simulink library "adrc_toolbox_library_2021"  (R2021a)
settings: Solver=VariableStepAuto  StartTime=0.0  StopTime=10.0  RelTol=1e-3
settings Model: Creator=krzys  LastModifiedBy=krzys

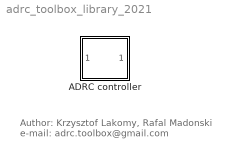
== system adrc_toolbox_library_2021 ==
  note: Author: Krzysztof Lakomy, Rafal Madonski
      | e-mail: adrc.toolbox@gmail.com
  ADRC controller : Subsystem  mask(ADRC controller){dynamicsOrder=2, controllerBandwidth=5, controllerBandwidthSource=Internal, observerBandwidth=25, observerBandwidthSource=Internal, inputGainParameter=1, inputGainSource=Internal, saturationEnabled=on, UpperLimit=10, LowerLimit=-10, deadTimeEnabled=off, deadTime=0.2}
      mask prompts: dynamicsOrder "Dynamics order (n):"; controllerBandwidth "Value [rad/s]:"; controllerBandwidthSource "Source:"; observerBandwidth "Value [rad/s]:"; observerBandwidthSource "Source:"; inputGainParameter "Value:"; inputGainSource "Source:"; saturationEnabled "Saturation"; UpperLimit "Upper limit (u_max):"; LowerLimit "Lower limit (u_min):"; deadTimeEnabled "Anti-peaking"; deadTime "Controller start time [s] (T_d):"
      mask help: The ADRC controller is a part of the Active Disturbance Rejection Control (ADRC) Toolbox, available at: https://www.mathworks.com/matlabcentral/fileexchange/102249-active-disturbance-rejection-control-adrc-toolbox
      mask init:
      | set_param(gcb,'MaskHideContents','off');
      | set_param(gcb, 'MaskSelfModifiable', 'on');
      | 
      | controllerBandwidthSource = get_param(gcb,'controllerBandwidthSource');
      | switch(controllerBandwidthSource)
      |     case 'Internal'
      |         replace_block([gcb,'/controllerBandwidthIn'], 'Inport', 'Ground', 'noprompt');
      |         inputGainParameterType = 'Internal';
      |     case 'External'
      |         replace_block([gcb,'/controllerBandwidthIn'], 'Ground', 'Inport', 'noprompt');
      |         inputGainParameterType = 'External';
      | end
      | 
      | observerBandwidthSource = get_param(gcb,'observerBandwidthSource');
      | switch(observerBandwidthSource)
      |     case 'Internal'
      |         replace_block([gcb,'/observerBandwidthIn'], 'Inport', 'Ground', 'noprompt');
      |         inputGainParameterType = 'Internal';
      |     case 'External'
      |         replace_block([gcb,'/observerBandwidthIn'], 'Ground', 'Inport', 'noprompt');
      |         inputGainParameterType = 'External';
      | end
      | 
      | inputGainSource = get_param(gcb,'inputGainSource');
      | switch(inputGainSource)
      |     case 'Internal'
      |         replace_block([gcb,'/inputGainParameterIn'], 'Inport', 'Ground', 'noprompt');
      |         inputGainParameterType = 'Internal';
      |     case 'External'
      |         replace_block([gcb,'/inputGainParameterIn'], 'Ground', 'Inport', 'noprompt');
      |         inputGainParameterType = 'External';
      | end
      mask Help:
      | The ADRC controller is a single, drag-and-drop, Simulink function block that encapsulates a specific continous-time error-based active disturbance rejection control (ADRC) algorithm. For simplicity and compactness, the ADRC controller is developed as a single input (feedback error signal), single output (control signal) block, which can be used as a powerful alternative to the conventional PID controller.
      | 
      | The design parameters of the implemented ADRC algorithm can be easily changed using the provided graphical user interface (GUI). The GUI also allows to activate two practical functionalities, namely: saturation of the control signal and anti-peaking mechanism.
      | 
      | The ADRC controller is a part of the Active Disturbance Rejection Control (ADRC) Toolbox. The goal of the Active Disturbance Rejection Control (ADRC) Toolbox is to provide an intuitive contol solution for Simulink, allowing to implement the ADRC algorithm in simulations/experiments quickly and with low effort.
      | 
      | Code contributors: Krzysztof Lakomy, Rafal Madonski, Jacek Michalski, Wojciech Giernacki
      | 
      | Contact: adrc.toolbox@gmail.com
      | 
      | More information at: https://www.mathworks.com/matlabcentral/fileexchange/102249-active-disturbance-rejection-control-adrc-toolbox
      mask TypeOptions dynamicsOrder: Linear extended state observer/dynamicsOrder | State feedback robust controller/dynamicsOrder
      mask TypeOptions controllerBandwidth: State feedback robust controller/controllerBandwidth
      mask TypeOptions controllerBandwidthSource: Internal | External
      mask Callback controllerBandwidthSource:
      | controllerBandwidthSource = get_param(gcb,'controllerBandwidthSource');
      | en = get_param(gcb,'MaskEnables');
      | 
      | switch(controllerBandwidthSource)
      |     case 'Internal'
      |         en{2} = 'on';
      |     case 'External'
      |         en{2} = 'off';
      | end
      | 
      | set_param(gcb,'MaskEnables',en);
      mask TypeOptions observerBandwidth: Linear extended state observer/observerBandwidth
      mask TypeOptions observerBandwidthSource: Internal | External
      mask Callback observerBandwidthSource:
      | observerBandwidthSource = get_param(gcb,'observerBandwidthSource');
      | en = get_param(gcb,'MaskEnables');
      | 
      | switch(observerBandwidthSource)
      |     case 'Internal'
      |         en{4} = 'on';
      |     case 'External'
      |         en{4} = 'off';
      | end
      | 
      | set_param(gcb,'MaskEnables',en);
      mask TypeOptions inputGainParameter: Linear extended state observer/inputGainParameter | State feedback robust controller/inputGainParameter
      mask TypeOptions inputGainSource: Internal | External
      mask Callback inputGainSource:
      | inputGainSource = get_param(gcb,'inputGainSource');
      | en = get_param(gcb,'MaskEnables');
      | 
      | switch(inputGainSource)
      |     case 'Internal'
      |         en{6} = 'on';
      |     case 'External'
      |         en{6} = 'off';
      | end
      | 
      | set_param(gcb,'MaskEnables',en);
      mask TypeOptions saturationEnabled: State feedback robust controller/saturationEnabled
      mask Callback saturationEnabled:
      | saturationEnabled = get_param(gcb,'saturationEnabled');
      | en = get_param(gcb,'MaskEnables');
      | 
      | switch(saturationEnabled)
      |     case 'on'
      |         en{9} = 'on';
      |         en{10} = 'on';
      |     case 'off'
      |         en{9} = 'off';
      |         en{10} = 'off';
      | end
      | 
      | set_param(gcb,'MaskEnables',en);
      mask TypeOptions UpperLimit: State feedback robust controller/UpperLimit
      mask TypeOptions LowerLimit: State feedback robust controller/LowerLimit
      mask TypeOptions deadTimeEnabled: State feedback robust controller/deadTimeEnabled
      mask Callback deadTimeEnabled:
      | deadTimeEnabled = get_param(gcb,'deadTimeEnabled');
      | en = get_param(gcb,'MaskEnables');
      | 
      | switch(deadTimeEnabled)
      |     case 'on'
      |         en{12} = 'on';
      |     case 'off'
      |         en{12} = 'off';
      | end
      | 
      | set_param(gcb,'MaskEnables',en);
      mask TypeOptions deadTime: State feedback robust controller/Time
      mask DialogControl DescGroupVar Prompt: Active Disturbance Rejection Controller (ADRC)
      mask DialogControl DescTextVar Prompt: This block implements an error-based continuous-time Active Disturbance Rejection Controller (ADRC). The default form of this controller calculates the control signal (block output) based only on the control feedback error (block input).
      mask DialogControl ParameterGroupVar Prompt: Control system parameters
      mask DialogControl Container5 Prompt: Parameters
      mask DialogControl Container12 Prompt: Controller bandwidth (omega_c):
      mask DialogControl Container11 Prompt: Observer bandwidth (omega_o):
      mask DialogControl Container10 Prompt: Input gain (b_hat):
      mask DialogControl Container4 Prompt: Saturation
      mask DialogControl Control3 Prompt: Saturation functionality limits the boundary values of the control signal, allowing to adjust the output of the ADRC controller block to the physical limitations of the controlled system.
      mask DialogControl Container8 Prompt: Anti-peaking
      mask DialogControl Control4 Prompt: Anti-peaking functionality is obtained by delaying the controller start by a specified time value (in seconds), allowing the observer transient state to pass.
      mask Display:
      | inputGainSource = get_param(gcb,'inputGainSource');
      | observerBandwidthSource = get_param(gcb,'observerBandwidthSource');
      | controllerBandwidthSource = get_param(gcb,'controllerBandwidthSource');
      | 
      | disp('ADRC');
      | switch controllerBandwidthSource
      |     case 'Internal'
      |     case 'External'
      |         port_label('input',1,'e');
      |         port_label('input',2,'wc');
      | end
      | switch observerBandwidthSource
      |     case 'Internal'
      |     case 'External'
      |         port_label('input',1,'e');
      |         if(strcmp(controllerBandwidthSource,'External'))
      |             port_label('input',3,'wo');
      |         else
      |             port_label('input',2,'wo');
      |         end
      | end
      | switch inputGainSource
      |     case 'Internal'
      |     case 'External'
      |         port_label('input',1,'e');
      |         if(strcmp(controllerBandwidthSource,'External') && strcmp(observerBandwidthSource,'External'))
      |             port_label('input',4,'b');
      |         elseif(xor(strcmp(controllerBandwidthSource,'External'), strcmp(observerBandwidthSource,'External')))
      |             port_label('input',3,'b');
      |         else
      |             port_label('input',2,'b');
      |         end
      | end

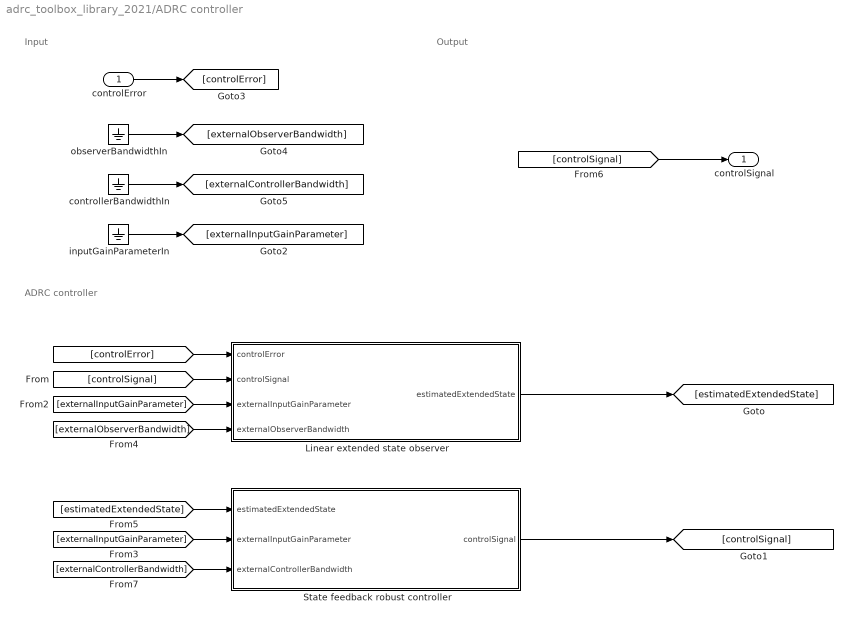
== system adrc_toolbox_library_2021/ADRC controller ==
  note: ADRC controller
  note: Output
  note: Input
  controlError : Inport
  Linear extended state observer : Subsystem  mask{InitialCondition=zeros(dynamicsOrder+1,1), dynamicsOrder=dynamicsOrder, observerBandwidth=observerBandwidth, inputGainParameter=inputGainParameter}
      mask prompts: InitialCondition "Integrator initial conditions:"; dynamicsOrder "Dynamics order:"; observerBandwidth "Observer bandwidth:"; inputGainParameter "Input gain parameter:"
      mask TypeOptions InitialCondition: Integrator/InitialCondition
      mask TypeOptions dynamicsOrder: Linear extended state observer/dynamicsOrder
      mask TypeOptions observerBandwidth: Linear extended state observer/observerBandwidth
      mask TypeOptions inputGainParameter: Linear extended state observer/inputGainParameter
  State feedback robust controller : Subsystem  mask{dynamicsOrder=dynamicsOrder, inputGainParameter=inputGainParameter, controllerBandwidth=controllerBandwidth, saturationEnabled=on, UpperLimit=UpperLimit, LowerLimit=LowerLimit, deadTimeEnabled=off, Time=deadTime}
      mask prompts: dynamicsOrder "Dynamics order:"; inputGainParameter "Input gain parameter:"; controllerBandwidth "Controller bandwidth:"; saturationEnabled "Output saturation"; UpperLimit "Simulink:blkprm_prompts:SaturateUpLim"; LowerLimit "Simulink:blkprm_prompts:SaturateLowLim"; deadTimeEnabled "Dead time enabled"; Time "Dead time:"
      mask TypeOptions dynamicsOrder: Extended state feedback robust controller/dynamicsOrder
      mask TypeOptions inputGainParameter: Extended state feedback robust controller/inputGainParameter
      mask TypeOptions controllerBandwidth: Extended state feedback robust controller/controllerBandwidth
      mask TypeOptions saturationEnabled: Saturation/saturationEnabled
      mask TypeOptions UpperLimit: Saturation/UpperLimit
      mask TypeOptions LowerLimit: Saturation/LowerLimit
      mask TypeOptions deadTimeEnabled: Dead time/deadTimeEnabled
      mask TypeOptions Time: Dead time/Time
      mask DialogControl UpperLimit Prompt: Upper limit:
      mask DialogControl LowerLimit Prompt: Lower limit:
  controllerBandwidthIn : Ground
  inputGainParameterIn : Ground
  observerBandwidthIn : Ground
  controlSignal : Outport
  wires:
  [controlSignal] -> controlSignal/1
  [controlError] -> Linear extended state observer/1(controlError)
  [controlSignal] -> Linear extended state observer/2(controlSignal)
  controlError/1 -> [controlError]
  Linear extended state observer/1(estimatedExtendedState) -> [estimatedExtendedState]
  [estimatedExtendedState] -> State feedback robust controller/1(estimatedExtendedState)
  inputGainParameterIn/1 -> [externalInputGainParameter]
  [externalInputGainParameter] -> Linear extended state observer/3(externalInputGainParameter)
  [externalInputGainParameter] -> State feedback robust controller/2(externalInputGainParameter)
  State feedback robust controller/1(controlSignal) -> [controlSignal]
  observerBandwidthIn/1 -> [externalObserverBandwidth]
  [externalObserverBandwidth] -> Linear extended state observer/4(externalObserverBandwidth)
  controllerBandwidthIn/1 -> [externalControllerBandwidth]
  [externalControllerBandwidth] -> State feedback robust controller/3(externalControllerBandwidth)

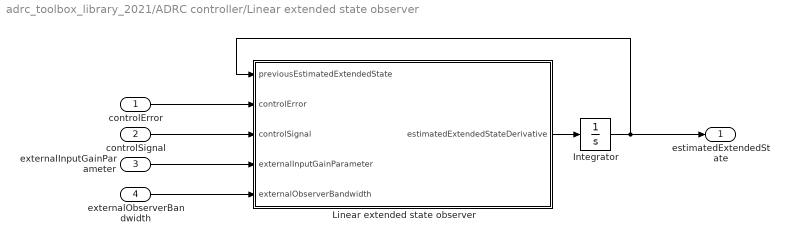
== system adrc_toolbox_library_2021/ADRC controller/Linear extended state observer ==
  controlError : Inport
  controlSignal : Inport  Port=2
  externalInputGainParameter : Inport  Port=3  PortDimensions=1
  externalObserverBandwidth : Inport  Port=4  PortDimensions=1
  Integrator : Integrator  InitialCondition=InitialCondition
  Linear extended state observer : MATLAB Function  TreatAsAtomicUnit=on  mask{dynamicsOrder=dynamicsOrder, observerBandwidth=observerBandwidth, inputGainParameter=inputGainParameter}
      mask prompts: dynamicsOrder "Dynamics order:"; observerBandwidth "Observer bandwidth:"; inputGainParameter "Input gain parameter:"
  estimatedExtendedState : Outport
  wires:
  controlError/1 -> Linear extended state observer/2(controlError)
  Linear extended state observer/1(estimatedExtendedStateDerivative) -> Integrator/1
  externalInputGainParameter/1 -> Linear extended state observer/4(externalInputGainParameter)
  controlSignal/1 -> Linear extended state observer/3(controlSignal)
  Integrator/1 -> Linear extended state observer/1(previousEstimatedExtendedState), estimatedExtendedState/1
  externalObserverBandwidth/1 -> Linear extended state observer/5(externalObserverBandwidth)

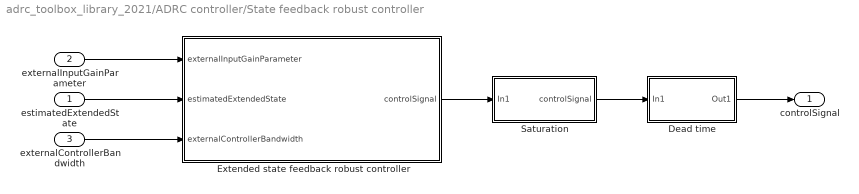
== system adrc_toolbox_library_2021/ADRC controller/State feedback robust controller ==
  estimatedExtendedState : Inport  PortDimensions=dynamicsOrder+1
  externalInputGainParameter : Inport  Port=2  PortDimensions=1  SampleTime=1
  externalControllerBandwidth : Inport  Port=3  PortDimensions=1
  Dead time : Subsystem  Variant=on  VariantControlMode=label  LabelModeActiveChoice=dead_time_off  mask{deadTimeEnabled=off, Time=Time}
      mask prompts: deadTimeEnabled "Dead time enabled"; Time "Dead time:"
      mask Callback deadTimeEnabled:
      | deadTimeChoice = get_param(gcb,'deadTimeEnabled');
      | if strcmp(deadTimeChoice,'off')
      |     set_param(gcb, 'LabelModeActiveChoice', 'dead_time_off');
      | else
      |     set_param(gcb, 'LabelModeActiveChoice', 'dead_time_on');
      | end
      mask TypeOptions Time: Dead time on/Step/Time
  Extended state feedback robust controller : MATLAB Function  TreatAsAtomicUnit=on  mask{dynamicsOrder=dynamicsOrder, inputGainParameter=inputGainParameter, controllerBandwidth=controllerBandwidth}
      mask prompts: dynamicsOrder "Dynamics order:"; inputGainParameter "Input gain parameter:"; controllerBandwidth "Controller bandwidth:"
  Saturation : Subsystem  Variant=on  VariantControlMode=label  LabelModeActiveChoice=saturation_off  mask{saturationEnabled=on, UpperLimit=UpperLimit, LowerLimit=LowerLimit}
      mask prompts: saturationEnabled "Output saturation"; UpperLimit "Simulink:blkprm_prompts:SaturateUpLim"; LowerLimit "Simulink:blkprm_prompts:SaturateLowLim"
      mask Callback saturationEnabled:
      | saturationChoice = get_param(gcb,'saturationEnabled');
      | if strcmp(saturationChoice,'off')
      |     set_param(gcb, 'LabelModeActiveChoice', 'saturation_off');
      | else
      |     set_param(gcb, 'LabelModeActiveChoice', 'saturation_on');
      | end
      mask TypeOptions UpperLimit: Saturation on/Saturation/UpperLimit
      mask TypeOptions LowerLimit: Saturation on/Saturation/LowerLimit
      mask DialogControl UpperLimit Prompt: Upper limit:
      mask DialogControl LowerLimit Prompt: Lower limit:
  controlSignal : Outport
  wires:
  estimatedExtendedState/1 -> Extended state feedback robust controller/2(estimatedExtendedState)
  externalInputGainParameter/1 -> Extended state feedback robust controller/1(externalInputGainParameter)
  Extended state feedback robust controller/1(controlSignal) -> Saturation/1(In1)
  externalControllerBandwidth/1 -> Extended state feedback robust controller/3(externalControllerBandwidth)
  Saturation/1(controlSignal) -> Dead time/1(In1)
  Dead time/1(Out1) -> controlSignal/1

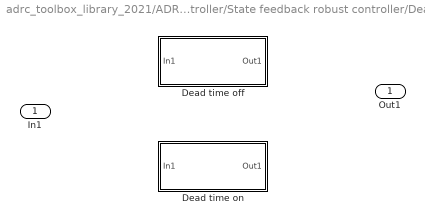
== system adrc_toolbox_library_2021/ADRC controller/State feedback robust controller/Dead time ==
  In1 : Inport
  Dead time off : Subsystem  VariantControl=dead_time_off
  Dead time on : Subsystem  VariantControl=dead_time_on
  Out1 : Outport

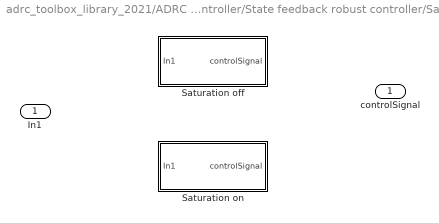
== system adrc_toolbox_library_2021/ADRC controller/State feedback robust controller/Saturation ==
  In1 : Inport
  Saturation off : Subsystem  VariantControl=saturation_off
  Saturation on : Subsystem  VariantControl=saturation_on
  controlSignal : Outport

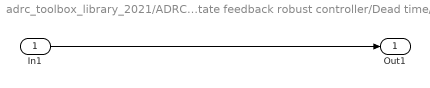
== system adrc_toolbox_library_2021/ADRC controller/State feedback robust controller/Dead time/Dead time off ==
  In1 : Inport
  Out1 : Outport
  wires:
  In1/1 -> Out1/1

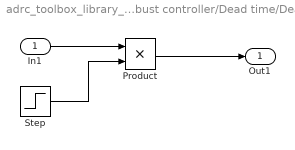
== system adrc_toolbox_library_2021/ADRC controller/State feedback robust controller/Dead time/Dead time on ==
  In1 : Inport
  Product : Product
  Step : Step  Time=Time  SampleTime=0
  Out1 : Outport
  wires:
  In1/1 -> Product/1
  Step/1 -> Product/2
  Product/1 -> Out1/1

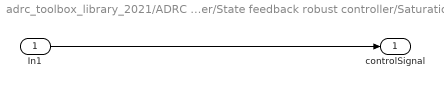
== system adrc_toolbox_library_2021/ADRC controller/State feedback robust controller/Saturation/Saturation off ==
  In1 : Inport
  controlSignal : Outport
  wires:
  In1/1 -> controlSignal/1

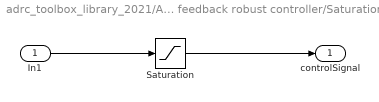
== system adrc_toolbox_library_2021/ADRC controller/State feedback robust controller/Saturation/Saturation on ==
  In1 : Inport
  Saturation : Saturate  UpperLimit=UpperLimit  LowerLimit=LowerLimit
  controlSignal : Outport
  wires:
  In1/1 -> Saturation/1
  Saturation/1 -> controlSignal/1

== matlab function adrc_toolbox_library_2021/ADRC controller/State feedback robust controller/Extended state feedback robust controller ==
  data: inputGainParameter parameter; externalInputGainParameter input; controllerBandwidth parameter; controlSignal output size=1; estimatedExtendedState input; externalControllerBandwidth input; dynamicsOrder parameter
function controlSignal = fcn(inputGainParameter,...
        externalInputGainParameter,...
        controllerBandwidth,...
        estimatedExtendedState,...
        externalControllerBandwidth,...
        dynamicsOrder)
    
    usedInputGain = evaluateSource(inputGainParameter, externalInputGainParameter);
    usedControllerBandwidth = evaluateSource(controllerBandwidth, externalControllerBandwidth);
    K = calculateControllerGain(usedControllerBandwidth, dynamicsOrder);
    
    controlSignal = 1/usedInputGain * (estimatedExtendedState(end) +...
            K * estimatedExtendedState(1:end-1));
end

function output = evaluateSource(internal, external)
    if(external == 0)
        output = internal;
    else
        output = external;
    end
end

function controllerGain = calculateControllerGain(controllerBandwidth, dynamicsOrder)
    extendedControllerGain = poly(-controllerBandwidth * ones(1, dynamicsOrder));
    controllerGain = flip(extendedControllerGain(2:end));
end

== matlab function adrc_toolbox_library_2021/ADRC controller/Linear extended state observer/Linear extended state observer ==
  data: previousEstimatedExtendedState input; controlError input; estimatedExtendedStateDerivative output; controlSignal input; dynamicsOrder parameter size=1; inputGainParameter parameter; externalInputGainParameter input; externalObserverBandwidth input; observerBandwidth parameter
function estimatedExtendedStateDerivative = fcn(previousEstimatedExtendedState,...
        controlError,...
        controlSignal,...
        dynamicsOrder,...
        inputGainParameter,...
        externalInputGainParameter,...
        externalObserverBandwidth,...
        observerBandwidth)
    
    usedInputGain = evaluateSource(inputGainParameter, externalInputGainParameter);
    usedObserverBandwidth = evaluateSource(observerBandwidth, externalObserverBandwidth);
    A = calculateObserverStateMatrix(dynamicsOrder);
    B = calculateObserverInputMatrix(usedInputGain, dynamicsOrder);
    L = calculateObserverGainVector(usedObserverBandwidth, dynamicsOrder);
    
    estimatedExtendedStateDerivative = A * previousEstimatedExtendedState +...
        B * controlSignal +...
        L * (controlError - previousEstimatedExtendedState(1));
end

function output = evaluateSource(internal, external)
    if(external == 0)
        output = internal;
    else
        output = external;
    end
end

function observerStateMatrix = calculateObserverStateMatrix(dynamicsOrder)
    observerStateMatrix = [zeros(dynamicsOrder,1), eye(dynamicsOrder);...
        zeros(1,dynamicsOrder+1)];
end

function observerInputMatrix = calculateObserverInputMatrix(inputGainParameter, dynamicsOrder)
    observerInputMatrix = [zeros(dynamicsOrder-1,1); -inputGainParameter; 0];
end

function observerGainVector = calculateObserverGainVector(observerBandwidth, dynamicsOrder)
    extendedGainVector = poly(-observerBandwidth * ones(1, dynamicsOrder+1))';
    observerGainVector = extendedGainVector(2:end);
end
